simulink model "DSM4"  (R2020a)
settings: Solver=VariableStepAuto  StartTime=0.0  StopTime=0.3  RelTol=1e-3
settings Model: Creator=bzhan  LastModifiedBy=bzhan

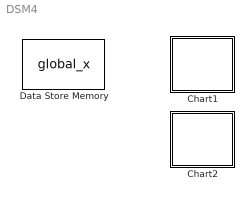
== system DSM4 ==
  Chart1 : Stateflow chart  TreatAsAtomicUnit=on
  Chart2 : Stateflow chart  TreatAsAtomicUnit=on
  Data Store Memory : DataStoreMemory  DataStoreName=global_x  ReadBeforeWriteMsg=warning  WriteAfterWriteMsg=warning  WriteAfterReadMsg=warning  InitialValue=1  ShowAdditionalParam=off  OutDataTypeStr=int32

== stateflow chart DSM4/Chart2 ==
  settings: updateMethod=DISCRETE  sampleTime=0.1
  state C
    en: f("C")
  state B
    en: f("D")
  (default) -> C
  C -> B : {global_x=global_x+2;}
  B -> C
  data: s function_input; global_x data_store_memory
  function f(s):
    | function f(s)
    |   fprintf(s+"%d\n", global_x);

== stateflow chart DSM4/Chart1 ==
  settings: updateMethod=DISCRETE  sampleTime=0.1
  state A
    en: f("A")
  state B
    en: f("B")
  (default) -> A
  A -> B : {global_x=global_x+1;}
  B -> A
  data: s function_input; global_x data_store_memory
  function f(s):
    | function f(s)
    |   fprintf(s+"%d\n", global_x);
